simulink model "Simulink_2gdl"  (R2020a)
settings: Solver=VariableStepAuto  StartTime=0.0  StopTime=720  RelTol=1e-3
libraries: dspsrcs4 x1
settings Model: Creator=Laura  LastModifiedBy=juan
settings SFSimCC: CustomCodeUndefinedFunction=UseInterfaceOnly

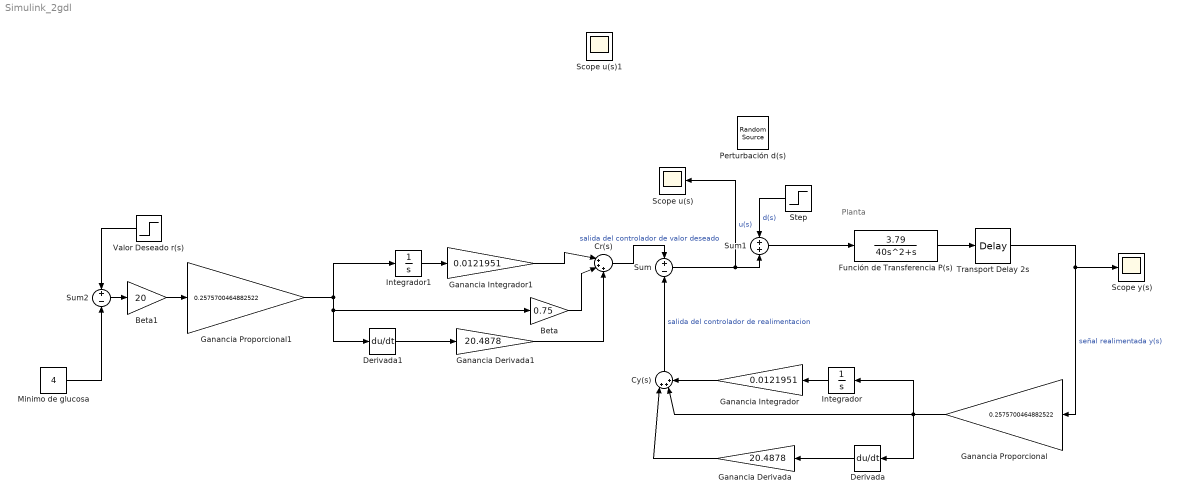
== system Simulink_2gdl ==
  note: Planta
  " Cr(s)" : Sum  Inputs=|+++
  " Cy(s)" : Sum  Inputs=|+++
  Beta : Gain  Gain=0.75
  Beta1 : Gain  Gain=20
  Derivada : Derivative
  Derivada1 : Derivative
  Función de Transferencia P(s) : TransferFcn  Numerator=[3.79]  Denominator=[40 1 0]
  Ganancia Derivada : Gain  Gain=20.4878
  Ganancia Derivada1 : Gain  Gain=20.4878
  Ganancia Integrador : Gain  Gain=0.0121951
  Ganancia Integrador1 : Gain  Gain=0.0121951
  Ganancia Proporcional : Gain  Gain=0.2575700464882522
  Ganancia Proporcional1 : Gain  Gain=0.2575700464882522
  Integrador : Integrator
  Integrador1 : Integrator
  Minimo de glucosa : Constant  Value=4
  "Perturbación d(s) " : dspsrcs4/Random Source  SrcType=Uniform  NormMethod=Ziggurat  CltLength=12  MinVal=0  MaxVal=1  MeanVal=0  VarVal=1  RepMode=Not repeatable  rawSeed=1  IsInherit=off  SampMode=Discrete  SampTime=1  SampFrame=1  DataType=Double  OutComplex=Real  OutputFrames=off
  Scope u(s) : Scope
  Scope u(s)1 : Scope
  Scope y(s) : Scope
  Step : Step  Time=360  After=20  SampleTime=0
  Sum : Sum  Inputs=+-
  Sum1 : Sum
  Sum2 : Sum  Inputs=+-
  Transport Delay 2s : TransportDelay  DelayTime=2
  Valor Deseado r(s) : Step  Time=180  Before=4.5  After=5.6  SampleTime=0
  wires:
  Integrador/1 -> Ganancia Integrador/1
  Derivada/1 -> Ganancia Derivada/1
  Ganancia Integrador/1 -> " Cy(s)"/3
  Ganancia Derivada/1 -> " Cy(s)"/1
  Función de Transferencia P(s)/1 -> Transport Delay 2s/1
  Ganancia Proporcional/1 -> " Cy(s)"/2, Integrador/1, Derivada/1
  Ganancia Proporcional1/1 -> Beta/1, Derivada1/1, Integrador1/1
  Integrador1/1 -> Ganancia Integrador1/1
  Derivada1/1 -> Ganancia Derivada1/1
  Ganancia Derivada1/1 -> " Cr(s)"/3
  Beta/1 -> " Cr(s)"/2
  Ganancia Integrador1/1 -> " Cr(s)"/1
  " Cr(s)"/1 -> Sum/1  "salida del controlador de valor deseado"
  " Cy(s)"/1 -> Sum/2  "salida del controlador de realimentacion"
  Sum/1 -> Scope u(s)/1, Sum1/2  "u(s)"
  Sum1/1 -> Función de Transferencia P(s)/1
  Transport Delay 2s/1 -> Scope y(s)/1, Ganancia Proporcional/1  "señal realimentada y(s)"
  Minimo de glucosa/1 -> Sum2/2
  Sum2/1 -> Beta1/1
  Beta1/1 -> Ganancia Proporcional1/1
  Valor Deseado r(s)/1 -> Sum2/1
  Step/1 -> Sum1/1  "d(s)"
